simulink model "untitled"  (R2017b)
settings: Solver=VariableStepAuto  StartTime=0.0  StopTime=10.0  RelTol=1e-3
libraries: neural x47
(part 4 of 4)

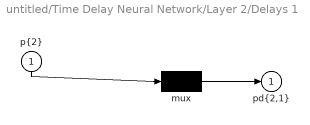
== system untitled/Time Delay Neural Network/Layer 2/Delays 1 ==
  "p{2}" : Inport  PortDimensions=42  SampleTime=1
      mask Display: e = 0.06;c1 = [120 230 180]/255;c2 = ([120 230 180]+0)/(256+128);c3 = ([120 230 180]+128)/(256+128);patch([0 1 1 0],[0 0 1 1],c1);patch([0 1 1 1-e 1-e 0+e],[0 0 1 1-e 0+e 0+e],c2);patch([0 0 1 1-e 0+e 0+e],[0 1 1 1-e 1-e 0+e],c3);plot([0 1 1 0 0],[0 0 1 1 0]);
  mux : Mux  Inputs=1
      mask Display: e = 0.06;c1 = [120 150 230]/255;c2 = ([120 150 230]+0)/383;c3 = ([120 150 230]+128)/383;patch([0 1 1 0],[0 0 1 1],c1);patch([0 1 1 1-e 1-e 0+e],[0 0 1 1-e 0+e 0+e],c2);patch([0 0 1 1-e 0+e 0+e],[0 1 1 1-e 1-e 0+e],c3);plot([0 1 1 0 0],[0 0 1 1 0]);disp('Mux')
  "pd{2,1}" : Outport
      mask Display: e = 0.06;c1 = [120 230 180]/255;c2 = ([120 230 180]+0)/(256+128);c3 = ([120 230 180]+128)/(256+128);patch([0 1 1 0],[0 0 1 1],c1);patch([0 1 1 1-e 1-e 0+e],[0 0 1 1-e 0+e 0+e],c2);patch([0 0 1 1-e 0+e 0+e],[0 1 1 1-e 1-e 0+e],c3);plot([0 1 1 0 0],[0 0 1 1 0]);
  wires:
  "p{2}"/1 -> mux/1
  mux/1 -> "pd{2,1}"/1

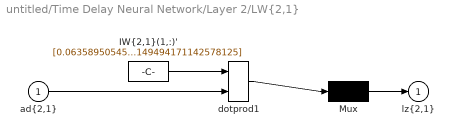
== system untitled/Time Delay Neural Network/Layer 2/LW{2,1} ==
  "ad{2,1}" : Inport  PortDimensions=42  SampleTime=1
      mask Display: e = 0.06;c1 = [120 230 180]/255;c2 = ([120 230 180]+0)/(256+128);c3 = ([120 230 180]+128)/(256+128);patch([0 1 1 0],[0 0 1 1],c1);patch([0 1 1 1-e 1-e 0+e],[0 0 1 1-e 0+e 0+e],c2);patch([0 0 1 1-e 0+e 0+e],[0 1 1 1-e 1-e 0+e],c3);plot([0 1 1 0 0],[0 0 1 1 0]);
  "IW{2,1}(1,:)'" : Constant  Value=[0.06358950545909845819547712153507745824754238128662109375;-0.06856844589833255287913971187663264572620391845703125;0.052249261880604892793744653545218170620501041412353515625;0.47566301053440873669586608230019919574260711669921875;-0.041836536715406137665329566743821487762033939361572265625;-0.047508097288857749351809189874984440393745899200439453125;-0.7238836614026933347076919744722545146942138671875;-0.0474282122725623589420962389340274967253208160400390625;0.42514409026680854974955536818015389144420623779296875;0.58523680569008751373161203446215949952602386474609375;0.370172859381687924251735921643557958304882049560546875;-0.049001286497569428168841199067173874936997890472412109375;0.002779864278295297343179814930635984637774527072906494140625;-0.06979973931064385739286848320261924527585506439208984375;0.056333084579634463973096814015661948360502719879150390625;-0.0682344775999774721952917388989590108394622802734375;0.06004882589342373788721118899047723971307277679443359375;-0.062011619477233055619525003976377774961292743682861328125;-0.0711344088632489268686498462557210586965084075927734375;-0.0641524993861022352348300046287477016448974609375;-0.5013411174553825677691065720864571630954742431640625;0.055191158594875937282164812813789467327296733856201171875;0.04713555683415317221207629927448579110205173492431640625;0.060916725691791899499616391722156549803912639617919921875;-0.07383218155751451738932900070722098462283611297607421875;-0.62519170934624934687917630071751773357391357421875;-0.315537027394343194686143760918639600276947021484375;0.05365016333487877819852229777097818441689014434814453125;0.0173407261737775313104048535706169786863029003143310546875;-0.047431328368500967618270891534848487935960292816162109375;-0.057013280386601063176588155556601122952997684478759765625;-0.0668563242167229676571338359281071461737155914306640625;-0.044860462713854555583115057970644556917250156402587890625;-0.0458105851155269638841360801961855031549930572509765625;-0.06060823829323082334585848229835391975939273834228515625;-0.039442283089036266063853730656774132512509822845458984375;-0.0405694180967702544560182786881341598927974700927734375;0.47998208196844005524184240130125544965267181396484375;-0.061477043636814894533859643388495896942913532257080078125;-0.06374082699332193902019838560590869747102260589599609375;0.44243348732659792954535760145517997443675994873046875;-0.0697568355994198363578817634333972819149494171142578125]
      mask Display: e = 0.06;c1 = [120 150 230]/255;c2 = ([120 150 230]+0)/383;c3 = ([120 150 230]+128)/383;patch([0 1 1 0],[0 0 1 1],c1);patch([0 1 1 1-e 1-e 0+e],[0 0 1 1-e 0+e 0+e],c2);patch([0 0 1 1-e 0+e 0+e],[0 1 1 1-e 1-e 0+e],c3);plot([0 1 1 0 0],[0 0 1 1 0]);disp('weights');
  Mux : Mux  Inputs=1
      mask Display: e = 0.06;c1 = [120 150 230]/255;c2 = ([120 150 230]+0)/383;c3 = ([120 150 230]+128)/383;patch([0 1 1 0],[0 0 1 1],c1);patch([0 1 1 1-e 1-e 0+e],[0 0 1 1-e 0+e 0+e],c2);patch([0 0 1 1-e 0+e 0+e],[0 1 1 1-e 1-e 0+e],c3);plot([0 1 1 0 0],[0 0 1 1 0]);disp('Mux');
  dotprod1 : neural/Weight Functions/dotprod
  "lz{2,1}" : Outport
      mask Display: e = 0.06;c1 = [120 230 180]/255;c2 = ([120 230 180]+0)/(256+128);c3 = ([120 230 180]+128)/(256+128);patch([0 1 1 0],[0 0 1 1],c1);patch([0 1 1 1-e 1-e 0+e],[0 0 1 1-e 0+e 0+e],c2);patch([0 0 1 1-e 0+e 0+e],[0 1 1 1-e 1-e 0+e],c3);plot([0 1 1 0 0],[0 0 1 1 0]);
  wires:
  "IW{2,1}(1,:)'"/1 -> dotprod1/1
  "ad{2,1}"/1 -> dotprod1/2
  dotprod1/1 -> Mux/1
  Mux/1 -> "lz{2,1}"/1
